simulink model "PercobaanMotorDC"  (R2014a)
settings: Solver=ode3  StartTime=0.0  StopTime=30  FixedStep=0.1  RelTol=1e-3
libraries: arduino_io_lib x4
settings Model: Creator=Lenovo  LastModifiedBy=Lenovo

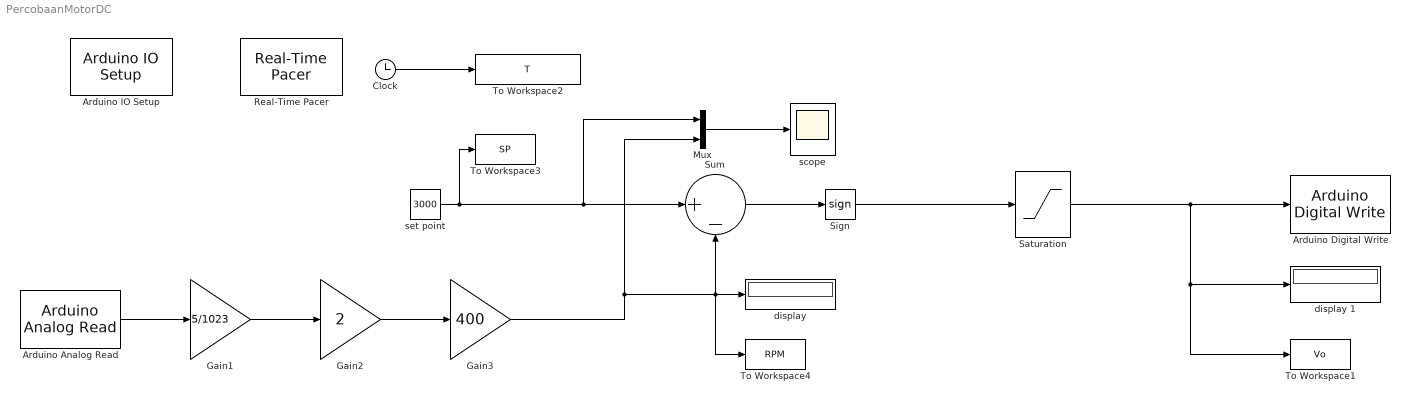
== system PercobaanMotorDC ==
  Arduino Analog Read : arduino_io_lib/Arduino Analog Read  arduinoVar=Temporary arduino variable: Arduino1  arduinoPin=0  T=0.1
  Arduino Digital Write : arduino_io_lib/Arduino Digital Write  arduinoVar=Temporary arduino variable: Arduino1  arduinoPin=3  T=0.1
  Arduino IO Setup : arduino_io_lib/Arduino IO Setup  Priority=3  arduinoVar=Temporary arduino variable: Arduino1  workspaceVarName=a  comPort=COM6
  Clock : Clock
  Gain1 : Gain  Gain=5/1023
  Gain2 : Gain  Gain=2
  Gain3 : Gain  Gain=400
  Mux : Mux  Inputs=2
  Real-Time Pacer : arduino_io_lib/Real-Time Pacer  simTimePerRealTime=1
  Saturation : Saturate  UpperLimit=1  LowerLimit=0
  Sign : Signum
  Sum : Sum  Inputs=|+-
  To Workspace1 : ToWorkspace  VariableName=Vo  SampleTime=-1
  To Workspace2 : ToWorkspace  VariableName=T  SampleTime=-1
  To Workspace3 : ToWorkspace  VariableName=SP  SampleTime=-1
  To Workspace4 : ToWorkspace  VariableName=RPM  SampleTime=-1
  "display " : Display
  display 1 : Display
  scope : Scope
      settings: YMin=2550  YMax=3100
  set point : Constant  Value=3000
  wires:
  Clock/1 -> To Workspace2/1
  Arduino Analog Read/1 -> Gain1/1
  Sign/1 -> Saturation/1
  Sum/1 -> Sign/1
  Gain1/1 -> Gain2/1
  Gain2/1 -> Gain3/1
  Mux/1 -> scope/1
  set point/1 -> To Workspace3/1, Mux/1, Sum/1
  Saturation/1 -> display 1/1, To Workspace1/1, Arduino Digital Write/1
  Gain3/1 -> To Workspace4/1, Sum/2, "display "/1, Mux/2
